simulink model "InductionMotorDynamicModelling"  (R2024a)
settings: Solver=ode23tb  StartTime=0.0  StopTime=1  FixedStep=1e-5  EnableMultiTasking=on
undefined symbols (not defined in the file): J, p, Rr, Rs, wb, Xlr, Xls, Xmstar
libraries: spsPLLLib x1, spsdq0toabcLib x1
settings Model: Creator=kavita  LastModifiedBy=danielmcguiness
settings SolverCC: MaxConsecutiveZCs=1  ZeroCrossAlgorithm=Adaptive  AlgebraicLoopSolver=TrustRegion
settings DataIOCC: LimitDataPoints=on  SaveFormat=Array  SignalLoggingSaveFormat=ModelDataLogs  ReturnWorkspaceOutputs=off
settings OptimizationCC: ExpressionDepthLimit=2147483647  LifeSpan=inf
settings DebuggingCC: UnderspecifiedInitializationDetection=Classic  MergeDetectMultiDrivingBlocksExec=none  SolverPrmCheckMsg=warning  FcnCallInpInsideContextMsg=warning  UnconnectedInputMsg=warning  UnconnectedOutputMsg=warning  UnconnectedLineMsg=warning  StateNameClashWarn=warning  SFUnexpectedBacktrackingDiag=warning  SFNoUnconditionalDefaultTransitionDiag=warning  SFExecutionAtInitializationDiag=none  ArithmeticOperatorsInVariantConditions=warning
settings HardwareCC: ProdBitPerPointer=32  ProdBitPerSizeT=32  ProdBitPerPtrDiffT=32  ProdLargestAtomicFloat=None  ProdIntDivRoundTo=Undefined  ProdEndianess=Unspecified  ProdWordSize=32  ProdHWDeviceType=32-bit Generic
settings ModelReferenceCC: EnableRefExpFcnMdlSchedulingChecks=on  PropagateSignalLabelsOutOfModel=off
settings SFSimCC: SimUseLocalCustomCode=off  CustomCodeUndefinedFunction=UseInterfaceOnly
settings RTWCC: RTWUseLocalCustomCode=off  GPUComputeCapability=3.5
settings CodeAppCC: StateflowObjectComments=on
settings GRTTargetCC: TargetLangStandard=C89/C90 (ANSI)  CombineOutputUpdateFcns=off  GRTInterface=on
settings ConfigComp: CovMetricSettings=dw  CovSaveCumulativeToWorkspaceVar=on  CovSaveSingleToWorkspaceVar=on  CovExternalEMLEnable=off

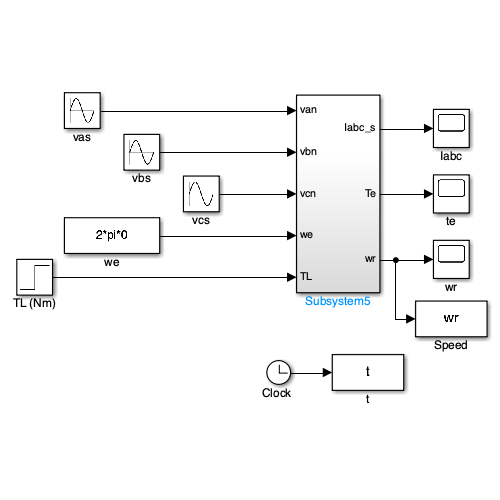
[thumbnail: Simulink's stored preview of the top-level diagram]
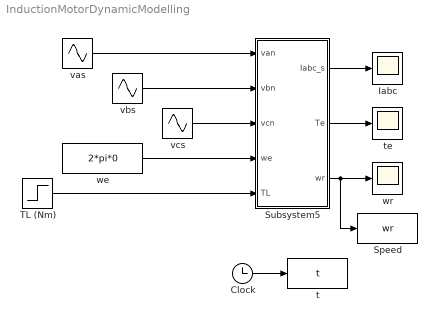
== system InductionMotorDynamicModelling ==
  "Clock " : Clock
  Iabc : Scope
  Speed : ToWorkspace  VariableName=wr  SaveFormat=Timeseries  SampleTime=-1
  Subsystem5 : Subsystem
  TL (Nm) : Step  Time=0.3  After=40  SampleTime=0
  t : ToWorkspace  VariableName=t  SaveFormat=Timeseries  SampleTime=-1
  te : Scope
  vas : Sin  Amplitude=200  Frequency=2*pi*50  SampleTime=0
  vbs : Sin  Amplitude=200  Frequency=2*pi*50  Phase=-120*pi/180  SampleTime=0
  vcs : Sin  Amplitude=200  Frequency=2*pi*50  Phase=-240*pi/180  SampleTime=0
  we : Constant  Value=2*pi*0
  wr : Scope
  wires:
  vas/1 -> Subsystem5/1(van)
  vbs/1 -> Subsystem5/2(vbn)
  vcs/1 -> Subsystem5/3(vcn)
  we/1 -> Subsystem5/4(we)
  TL (Nm)/1 -> Subsystem5/5(TL)
  Subsystem5/2(Te) -> te/1
  Subsystem5/3(wr) -> wr/1, Speed/1
  "Clock "/1 -> t/1
  Subsystem5/1(Iabc_s) -> Iabc/1

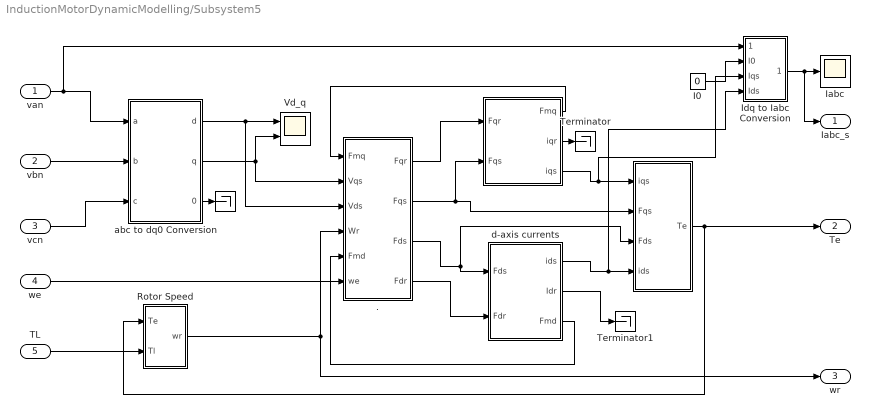
== system InductionMotorDynamicModelling/Subsystem5 ==
  van : Inport
  vbn : Inport  Port=2
  vcn : Inport  Port=3
  we : Inport  Port=4
  TL : Inport  Port=5
  " " : Subsystem
  "  " : Subsystem
  "            " : Terminator
  . : Subsystem
  I0 : Constant  Value=0
  Iabc : Scope
  Idq to Iabc Conversion : Subsystem
  Rotor Speed : Subsystem
  Terminator : Terminator
  Terminator1 : Terminator
  Vd_q : Scope  NumInputPorts=2
  abc to dq0 Conversion : Subsystem
  d-axis currents : Subsystem
  Iabc_s : Outport  VectorParamsAs1DForOutWhenUnconnected=off
  Te : Outport  Port=2  VectorParamsAs1DForOutWhenUnconnected=off
  wr : Outport  Port=3  VectorParamsAs1DForOutWhenUnconnected=off
  wires:
  " "/1(Te) -> Te/1, Rotor Speed/1(Te)
  abc to dq0 Conversion/2(q) -> ./2(Vqs), Vd_q/2
  abc to dq0 Conversion/1(d) -> ./3(Vds), Vd_q/1
  abc to dq0 Conversion/3(0) -> "            "/1
  vbn/1 -> abc to dq0 Conversion/2(b)
  ./2(Fqs) -> " "/2(Fqs), "  "/2(Fqs)
  ./4(Fdr) -> d-axis currents/2(Fdr)
  ./1(Fqr) -> "  "/1(Fqr)
  ./3(Fds) -> d-axis currents/1(Fds), " "/3(Fds)
  vcn/1 -> abc to dq0 Conversion/3(c)
  TL/1 -> Rotor Speed/2(Tl)
  "  "/1(Fmq) -> ./1(Fmq)
  we/1 -> ./6(we)
  Rotor Speed/1(wr) -> wr/1, ./4(Wr)
  d-axis currents/2(Idr) -> Terminator1/1
  d-axis currents/1(ids) -> Idq to Iabc Conversion/4(Ids), " "/4(ids)
  d-axis currents/3(Fmd) -> ./5(Fmd)
  "  "/2(iqr) -> Terminator/1
  "  "/3(iqs) -> Idq to Iabc Conversion/3(Iqs), " "/1(iqs)
  van/1 -> Idq to Iabc Conversion/1(van), abc to dq0 Conversion/1(a)
  I0/1 -> Idq to Iabc Conversion/2(I0)
  Idq to Iabc Conversion/1(Iabc) -> Iabc/1, Iabc_s/1

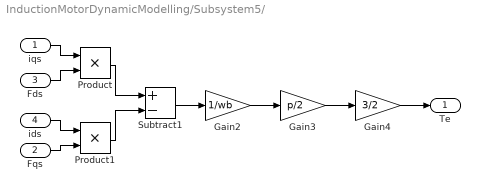
== system InductionMotorDynamicModelling/Subsystem5/  ==
  iqs : Inport
  Fqs : Inport  Port=2
  Fds : Inport  Port=3
  ids : Inport  Port=4
  Gain2 : Gain  Gain=1/wb
  Gain3 : Gain  Gain=p/2
  Gain4 : Gain  Gain=3/2
  Product : Product  RndMeth=Zero
  Product1 : Product  RndMeth=Zero
  Subtract1 : Sum  Inputs=+-
  Te : Outport  VectorParamsAs1DForOutWhenUnconnected=off
  wires:
  Gain4/1 -> Te/1
  Gain3/1 -> Gain4/1
  Gain2/1 -> Gain3/1
  Subtract1/1 -> Gain2/1
  Product1/1 -> Subtract1/2
  Product/1 -> Subtract1/1
  Fqs/1 -> Product1/2
  ids/1 -> Product1/1
  Fds/1 -> Product/2
  iqs/1 -> Product/1

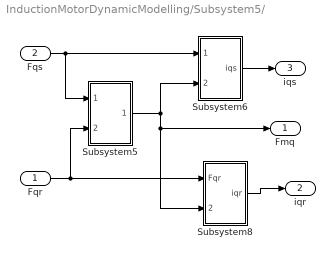
== system InductionMotorDynamicModelling/Subsystem5/   ==
  Fqr : Inport
  Fqs : Inport  Port=2
  Subsystem5 : Subsystem
  Subsystem6 : Subsystem
  Subsystem8 : Subsystem
  Fmq : Outport  VectorParamsAs1DForOutWhenUnconnected=off
  iqr : Outport  Port=2  VectorParamsAs1DForOutWhenUnconnected=off
  iqs : Outport  Port=3  VectorParamsAs1DForOutWhenUnconnected=off
  wires:
  Subsystem5/1(Fmq) -> Subsystem8/2(Fmq), Fmq/1, Subsystem6/2(Fmq)
  Fqs/1 -> Subsystem6/1(Fqs), Subsystem5/1(Fqs)
  Fqr/1 -> Subsystem8/1(Fqr), Subsystem5/2(Fqr)
  Subsystem6/1(iqs) -> iqs/1
  Subsystem8/1(iqr) -> iqr/1

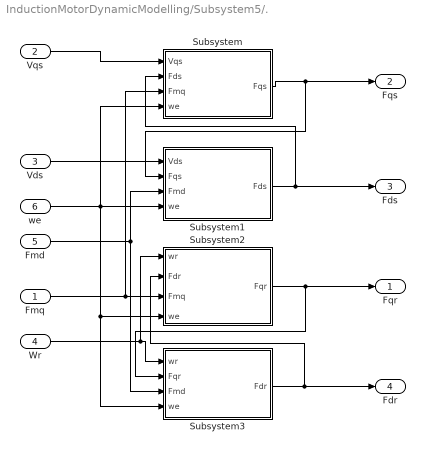
== system InductionMotorDynamicModelling/Subsystem5/. ==
  Fmq : Inport
  Vqs : Inport  Port=2
  Vds : Inport  Port=3
  Wr : Inport  Port=4
  Fmd : Inport  Port=5
  we : Inport  Port=6
  Subsystem : Subsystem
  Subsystem1 : Subsystem
  Subsystem2 : Subsystem
  Subsystem3 : Subsystem
  Fqr : Outport  VectorParamsAs1DForOutWhenUnconnected=off
  Fqs : Outport  Port=2  VectorParamsAs1DForOutWhenUnconnected=off
  Fds : Outport  Port=3  VectorParamsAs1DForOutWhenUnconnected=off
  Fdr : Outport  Port=4  VectorParamsAs1DForOutWhenUnconnected=off
  wires:
  Subsystem3/1(Fdr) -> Fdr/1, Subsystem2/2(Fdr)
  Subsystem2/1(Fqr) -> Subsystem3/2(Fqr), Fqr/1
  Subsystem/1(Fqs) -> Subsystem1/2(Fqs), Fqs/1
  Subsystem1/1(Fds) -> Subsystem/2(Fds), Fds/1
  Vqs/1 -> Subsystem/1(Vqs)
  Vds/1 -> Subsystem1/1(Vds)
  Fmd/1 -> Subsystem1/3(Fmd), Subsystem3/3(Fmd)
  Fmq/1 -> Subsystem2/3(Fmq), Subsystem/3(Fmq)
  Wr/1 -> Subsystem3/1(wr), Subsystem2/1(wr)
  we/1 -> Subsystem3/4(we), Subsystem2/4(we), Subsystem1/4(we), Subsystem/4(we)

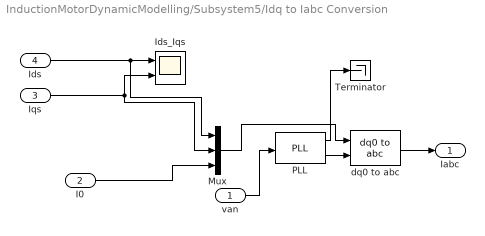
== system InductionMotorDynamicModelling/Subsystem5/Idq to Iabc Conversion ==
  van : Inport
  I0 : Inport  Port=2
  Iqs : Inport  Port=3
  Ids : Inport  Port=4
  Ids_Iqs : Scope  NumInputPorts=2
  Mux : Mux  Inputs=3
  PLL : spsPLLLib/PLL  Fmin=50  Par_Init=[0, 60]  ParK=[180, 3200, 1]  TcD=1e-4  MaxRateChangeFreq=12  FilterCutOffFreq=25  Ts=0  AGC=on
      settings: LibrarySourceBlock=sps_lib/Control/PLL
  Terminator : Terminator
  dq0 to abc : spsdq0toabcLib/dq0 to abc  Alignment=90 degrees behind phase A axis
  Iabc : Outport  VectorParamsAs1DForOutWhenUnconnected=off
  wires:
  van/1 -> PLL/1
  PLL/2 -> dq0 to abc/2
  I0/1 -> Mux/3
  Iqs/1 -> Ids_Iqs/2, Mux/2
  Ids/1 -> Mux/1, Ids_Iqs/1
  PLL/1 -> Terminator/1
  Mux/1 -> dq0 to abc/1
  dq0 to abc/1 -> Iabc/1

== system InductionMotorDynamicModelling/Subsystem5/Rotor Speed ==
  Te : Inport
  Tl : Inport  Port=2
  Gain1 : Gain  Gain=1/J
  Gain2 : Gain  Gain=p/2
  Integrator : Integrator
  Subtract : Sum  Inputs=+-
  wr : Outport  VectorParamsAs1DForOutWhenUnconnected=off
  wires:
  Te/1 -> Subtract/1
  Gain1/1 -> Gain2/1
  Subtract/1 -> Gain1/1
  Gain2/1 -> Integrator/1
  Integrator/1 -> wr/1
  Tl/1 -> Subtract/2

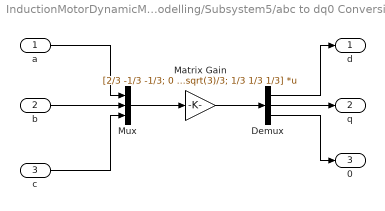
== system InductionMotorDynamicModelling/Subsystem5/abc to dq0 Conversion ==
  a : Inport
  b : Inport  Port=2
  c : Inport  Port=3
  Demux : Demux  Outputs=3
  Matrix Gain : Gain  Gain=[2/3 -1/3 -1/3; 0 sqrt(3)/3 -sqrt(3)/3; 1/3 1/3 1/3]  Multiplication=Matrix(K*u)  SaturateOnIntegerOverflow=on  OutDataTypeStr=Inherit: Same as input  ParamDataTypeStr=Inherit: Same as input
  Mux : Mux  Inputs=3
  d : Outport  VectorParamsAs1DForOutWhenUnconnected=off
  q : Outport  Port=2  VectorParamsAs1DForOutWhenUnconnected=off
  0 : Outport  Port=3  VectorParamsAs1DForOutWhenUnconnected=off
  wires:
  a/1 -> Mux/1
  b/1 -> Mux/2
  c/1 -> Mux/3
  Demux/1 -> d/1
  Demux/2 -> q/1
  Demux/3 -> 0/1
  Mux/1 -> Matrix Gain/1
  Matrix Gain/1 -> Demux/1

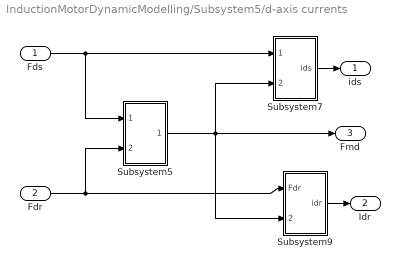
== system InductionMotorDynamicModelling/Subsystem5/d-axis currents ==
  Fds : Inport
  Fdr : Inport  Port=2
  Subsystem5 : Subsystem
  Subsystem7 : Subsystem
  Subsystem9 : Subsystem
  ids : Outport  VectorParamsAs1DForOutWhenUnconnected=off
  Idr : Outport  Port=2  VectorParamsAs1DForOutWhenUnconnected=off
  Fmd : Outport  Port=3  VectorParamsAs1DForOutWhenUnconnected=off
  wires:
  Subsystem5/1(Fmd) -> Subsystem7/2(Fmd), Subsystem9/2(Fmd), Fmd/1
  Fds/1 -> Subsystem7/1(Fds), Subsystem5/1(Fds)
  Fdr/1 -> Subsystem9/1(Fdr), Subsystem5/2(Fdr)
  Subsystem7/1(ids) -> ids/1
  Subsystem9/1(idr) -> Idr/1

== system InductionMotorDynamicModelling/Subsystem5/  /Subsystem5 ==
  Fqs : Inport
  Fqr : Inport  Port=2
  Fqr/Xlr : Gain  Gain=1/Xlr
  Fqs/Xls : Gain  Gain=1/Xls
  Gain : Gain  Gain=Xmstar
  Sum : Sum
  Fmq : Outport  VectorParamsAs1DForOutWhenUnconnected=off
  wires:
  Gain/1 -> Fmq/1
  Sum/1 -> Gain/1
  Fqr/1 -> Fqr/Xlr/1
  Fqs/1 -> Fqs/Xls/1
  Fqs/Xls/1 -> Sum/1
  Fqr/Xlr/1 -> Sum/2

== system InductionMotorDynamicModelling/Subsystem5/  /Subsystem6 ==
  Fqs : Inport
  Fmq : Inport  Port=2
  Gain : Gain  Gain=1/Xls
  Subtract : Sum  Inputs=+-
  iqs : Outport  VectorParamsAs1DForOutWhenUnconnected=off
  wires:
  Gain/1 -> iqs/1
  Subtract/1 -> Gain/1
  Fmq/1 -> Subtract/2
  Fqs/1 -> Subtract/1

== system InductionMotorDynamicModelling/Subsystem5/  /Subsystem8 ==
  Fqr : Inport
  Fmq : Inport  Port=2
  Gain : Gain  Gain=1/Xlr
  Subtract : Sum  Inputs=+-
  iqr : Outport  VectorParamsAs1DForOutWhenUnconnected=off
  wires:
  Subtract/1 -> Gain/1
  Fqr/1 -> Subtract/1
  Fmq/1 -> Subtract/2
  Gain/1 -> iqr/1

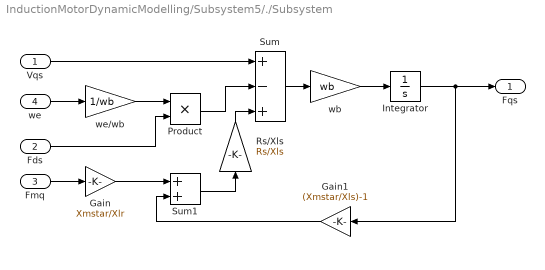
== system InductionMotorDynamicModelling/Subsystem5/./Subsystem ==
  Vqs : Inport
  Fds : Inport  Port=2
  Fmq : Inport  Port=3
  we : Inport  Port=4
  Gain : Gain  Gain=Xmstar/Xlr
  Gain1 : Gain  Gain=(Xmstar/Xls)-1
  Integrator : Integrator
  Product : Product  RndMeth=Zero
  Rs/Xls : Gain  Gain=Rs/Xls
  Sum : Sum  Inputs=+-+
  Sum1 : Sum
  wb : Gain  Gain=wb
  we/wb : Gain  Gain=1/wb
  Fqs : Outport  VectorParamsAs1DForOutWhenUnconnected=off
  wires:
  Vqs/1 -> Sum/1
  we/1 -> we/wb/1
  we/wb/1 -> Product/1
  Fds/1 -> Product/2
  Product/1 -> Sum/2
  Sum/1 -> wb/1
  wb/1 -> Integrator/1
  Integrator/1 -> Fqs/1, Gain1/1
  Fmq/1 -> Gain/1
  Rs/Xls/1 -> Sum/3
  Sum1/1 -> Rs/Xls/1
  Gain/1 -> Sum1/1
  Gain1/1 -> Sum1/2

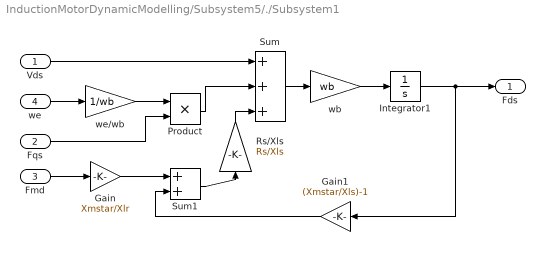
== system InductionMotorDynamicModelling/Subsystem5/./Subsystem1 ==
  Vds : Inport
  Fqs : Inport  Port=2
  Fmd : Inport  Port=3
  we : Inport  Port=4
  Gain : Gain  Gain=Xmstar/Xlr
  Gain1 : Gain  Gain=(Xmstar/Xls)-1
  Integrator1 : Integrator
  Product : Product  RndMeth=Zero
  Rs/Xls : Gain  Gain=Rs/Xls
  Sum : Sum  Inputs=+++
  Sum1 : Sum
  wb : Gain  Gain=wb
  we/wb : Gain  Gain=1/wb
  Fds : Outport  VectorParamsAs1DForOutWhenUnconnected=off
  wires:
  Sum1/1 -> Rs/Xls/1
  Rs/Xls/1 -> Sum/3
  Fmd/1 -> Gain/1
  Integrator1/1 -> Fds/1, Gain1/1
  wb/1 -> Integrator1/1
  Sum/1 -> wb/1
  Product/1 -> Sum/2
  Fqs/1 -> Product/2
  we/wb/1 -> Product/1
  we/1 -> we/wb/1
  Vds/1 -> Sum/1
  Gain/1 -> Sum1/1
  Gain1/1 -> Sum1/2

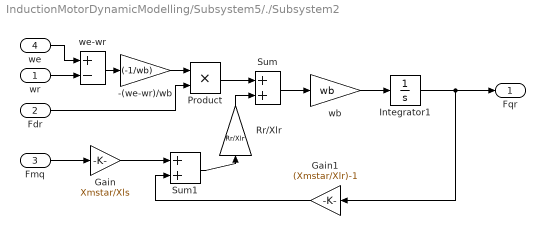
== system InductionMotorDynamicModelling/Subsystem5/./Subsystem2 ==
  wr : Inport
  Fdr : Inport  Port=2
  Fmq : Inport  Port=3
  we : Inport  Port=4
  -(we-wr)/wb : Gain  Gain=(-1/wb)
  Gain : Gain  Gain=Xmstar/Xls
  Gain1 : Gain  Gain=(Xmstar/Xlr)-1
  Integrator1 : Integrator
  Product : Product  RndMeth=Zero
  Rr/Xlr : Gain  Gain=Rr/Xlr
  Sum : Sum
  Sum1 : Sum
  wb : Gain  Gain=wb
  we-wr : Sum  Inputs=+-
  Fqr : Outport  VectorParamsAs1DForOutWhenUnconnected=off
  wires:
  Sum/1 -> wb/1
  wb/1 -> Integrator1/1
  Integrator1/1 -> Fqr/1, Gain1/1
  Fmq/1 -> Gain/1
  Sum1/1 -> Rr/Xlr/1
  Rr/Xlr/1 -> Sum/2
  Product/1 -> Sum/1
  Fdr/1 -> Product/2
  -(we-wr)/wb/1 -> Product/1
  we-wr/1 -> -(we-wr)/wb/1
  we/1 -> we-wr/1
  wr/1 -> we-wr/2
  Gain/1 -> Sum1/1
  Gain1/1 -> Sum1/2

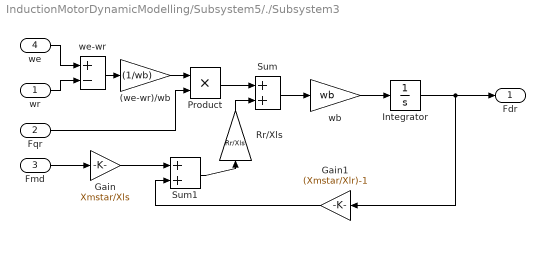
== system InductionMotorDynamicModelling/Subsystem5/./Subsystem3 ==
  wr : Inport
  Fqr : Inport  Port=2
  Fmd : Inport  Port=3
  we : Inport  Port=4
  (we-wr)/wb : Gain  Gain=(1/wb)
  Gain : Gain  Gain=Xmstar/Xls
  Gain1 : Gain  Gain=(Xmstar/Xlr)-1
  Integrator : Integrator
  Product : Product  RndMeth=Zero
  Rr/Xls : Gain  Gain=Rr/Xls
  Sum : Sum
  Sum1 : Sum
  wb : Gain  Gain=wb
  we-wr : Sum  Inputs=+-
  Fdr : Outport  VectorParamsAs1DForOutWhenUnconnected=off
  wires:
  wr/1 -> we-wr/2
  we/1 -> we-wr/1
  we-wr/1 -> (we-wr)/wb/1
  (we-wr)/wb/1 -> Product/1
  Fqr/1 -> Product/2
  Product/1 -> Sum/1
  Rr/Xls/1 -> Sum/2
  Sum1/1 -> Rr/Xls/1
  Fmd/1 -> Gain/1
  Integrator/1 -> Fdr/1, Gain1/1
  wb/1 -> Integrator/1
  Sum/1 -> wb/1
  Gain/1 -> Sum1/1
  Gain1/1 -> Sum1/2

== system InductionMotorDynamicModelling/Subsystem5/d-axis currents/Subsystem5 ==
  Fds : Inport
  Fdr : Inport  Port=2
  Fdr/Xlr : Gain  Gain=1/Xlr
  Fds/Xls : Gain  Gain=1/Xls
  Gain : Gain  Gain=Xmstar
  Sum : Sum
  Fmd : Outport  VectorParamsAs1DForOutWhenUnconnected=off
  wires:
  Gain/1 -> Fmd/1
  Sum/1 -> Gain/1
  Fdr/1 -> Fdr/Xlr/1
  Fds/1 -> Fds/Xls/1
  Fds/Xls/1 -> Sum/1
  Fdr/Xlr/1 -> Sum/2

== system InductionMotorDynamicModelling/Subsystem5/d-axis currents/Subsystem7 ==
  Fds : Inport
  Fmd : Inport  Port=2
  Gain : Gain  Gain=1/Xls
  Subtract : Sum  Inputs=+-
  ids : Outport  VectorParamsAs1DForOutWhenUnconnected=off
  wires:
  Subtract/1 -> Gain/1
  Fds/1 -> Subtract/1
  Fmd/1 -> Subtract/2
  Gain/1 -> ids/1

== system InductionMotorDynamicModelling/Subsystem5/d-axis currents/Subsystem9 ==
  Fdr : Inport
  Fmd : Inport  Port=2
  Gain : Gain  Gain=1/Xlr
  Subtract : Sum  Inputs=+-
  idr : Outport  VectorParamsAs1DForOutWhenUnconnected=off
  wires:
  Subtract/1 -> Gain/1
  Fdr/1 -> Subtract/1
  Fmd/1 -> Subtract/2
  Gain/1 -> idr/1
